simulink model "pwaSys_obs_model_ud"  (Simulink 8.6)
settings: Solver=ode45  StartTime=0.0  StopTime=sim_T  RelTol=1e-3
InitFcn:
  | load simulink.mat
  | setParameters
StartFcn:
  | load simulink.mat
  | setParameters
  | clear res_X res_U res_Y res_P res_D
  | clear res_Xest res_Dest res_Yest
StopFcn:
  | plotScope
undefined symbols (not defined in the file): sigbuilder_block, sim_A, sim_B, sim_C, sim_D, sim_d, sim_d_scale_bias, sim_d_scale_gain, sim_H, sim_K, sim_nx, sim_ny, sim_Ts, sim_u, sim_u_scale_bias, sim_u_scale_gain, sim_x0, sim_x_scale_bias, sim_x_scale_gain, sim_y_scale_bias, sim_y_scale_gain
libraries: xbsIndex_r4 x8
settings Model: Creator=alberto  LastModifiedBy=matteo
settings DataIOCC: SignalLoggingSaveFormat=Dataset
settings OptimizationCC: ExpressionDepthLimit=128
settings DebuggingCC: UnderspecifiedInitializationDetection=Simplified  MergeDetectMultiDrivingBlocksExec=error  FcnCallInpInsideContextMsg=EnableAllAsError  StateNameClashWarn=none
settings GRTTargetCC: CombineOutputUpdateFcns=on  GRTInterface=off
settings ConfigComp: CovSFcnEnable=off

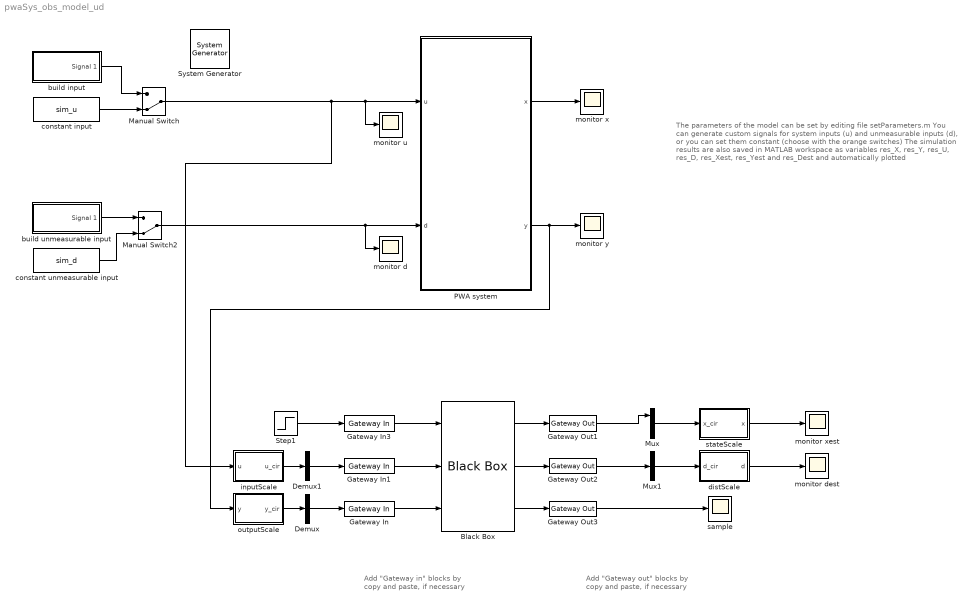
== system pwaSys_obs_model_ud ==
  note: The parameters of the model can be set by editing file setParameters.m
      |
      | You can generate custom signals for system inputs (u) and unmeasurable
      | inputs (d), or you can set them constant (choose with the orange switches)
      |
      | The simulation results are also saved in MATLAB workspace as variables
      | res_X, res_Y, res_U, res_D, res_Xest, res_Yest and res_Dest and
      | automatically plotted
  note: Add "Gateway out" blocks
      | by copy and paste,
      | if necessary
  note: Add "Gateway in" blocks
      | by copy and paste,
      | if necessary
  " System Generator" : xbsIndex_r4/ System Generator  Tag=genX  xilinxfamily=kintex7  part=xc7k325t  speed=-3  package=fbg676  synthesis_tool=Vivado  clock_wrapper=Clock Enables  directory=./netlist  proj_type=Vivado  Synth_file=Vivado Synthesis Defaults  Impl_file=Vivado Implementation Defaults  testbench=off  simulink_period=clk_period  sysclk_period=10  dcm_input_clock_period=10  incr_netlist=off  trim_vbits=Everywhere in SubSystem  dbl_ovrd=According to Block Masks  core_generation=According to Block Masks  run_coregen=off  deprecated_control=off  eval_field=0  block_type=sysgen
  Black Box : xbsIndex_r4/Black Box  init_code=embeddedSystem_config  sim_method=ISE Simulator  verbose=off  block_type=blackbox2
  Demux : Demux  Outputs=sim_ny
  Demux1 : Demux  Outputs=sim_nu
  Gateway In : xbsIndex_r4/Gateway In  gui_display_data_type=Fixed-point  arith_type="Signed  (2's comp)"  n_bits=sim_n_bit_in  bin_pt=0  preci_type=Single  exp_width=8  frac_width=24  rows=1  columns=1  quantization="Round  (unbiased: +/- Inf)"  overflow=Saturate  period=clk_period  UseAsADC=off  ADCChannel='1'  interface=None  automatic_assignment=on  address_offset=hex2dec('00')  intf_name=''  intf_description=''  timing_constraint=None  locs_specified=off  LOCs={}  io_standard={}  inherit_from_input=off  hdl_port=on  dbl_ovrd=off  block_type=gatewayin
  Gateway In1 : xbsIndex_r4/Gateway In  gui_display_data_type=Fixed-point  arith_type="Signed  (2's comp)"  n_bits=sim_n_bit_in  bin_pt=0  preci_type=Single  exp_width=8  frac_width=24  rows=1  columns=1  quantization="Round  (unbiased: +/- Inf)"  overflow=Saturate  period=clk_period  UseAsADC=off  ADCChannel='1'  interface=None  automatic_assignment=on  address_offset=hex2dec('00')  intf_name=''  intf_description=''  timing_constraint=None  locs_specified=off  LOCs={}  io_standard={}  inherit_from_input=off  hdl_port=on  dbl_ovrd=off  block_type=gatewayin
  Gateway In3 : xbsIndex_r4/Gateway In  gui_display_data_type=Boolean  arith_type=Boolean  n_bits=16  bin_pt=14  preci_type=Single  exp_width=8  frac_width=24  rows=1  columns=1  quantization="Round  (unbiased: +/- Inf)"  overflow=Saturate  period=clk_period  UseAsADC=off  ADCChannel='1'  interface=None  automatic_assignment=on  address_offset=hex2dec('00')  intf_name=''  intf_description=''  timing_constraint=None  locs_specified=off  LOCs={}  io_standard={}  inherit_from_input=off  hdl_port=on  dbl_ovrd=off  block_type=gatewayin
  Gateway Out1 : xbsIndex_r4/Gateway Out  inherit_from_input=off  hdl_port=on  rows=1  columns=1  UseAsDAC=off  DACChannel='1'  interface=None  automatic_assignment=on  address_offset=hex2dec('00')  intf_name=''  intf_description=''  timing_constraint=None  locs_specified=off  LOCs={}  io_standard={}  block_type=gatewayout
  Gateway Out2 : xbsIndex_r4/Gateway Out  inherit_from_input=off  hdl_port=on  rows=1  columns=1  UseAsDAC=off  DACChannel='1'  interface=None  automatic_assignment=on  address_offset=hex2dec('00')  intf_name=''  intf_description=''  timing_constraint=None  locs_specified=off  LOCs={}  io_standard={}  block_type=gatewayout
  Gateway Out3 : xbsIndex_r4/Gateway Out  inherit_from_input=off  hdl_port=on  rows=1  columns=1  UseAsDAC=off  DACChannel='1'  interface=None  automatic_assignment=on  address_offset=hex2dec('00')  intf_name=''  intf_description=''  timing_constraint=None  locs_specified=off  LOCs={}  io_standard={}  block_type=gatewayout
  Manual Switch : ManualSwitch  CurrentSetting=0
  Manual Switch2 : ManualSwitch  CurrentSetting=0
  Mux : Mux  Inputs=sim_nx
  Mux1 : Mux  Inputs=sim_nd
  PWA system : Subsystem
  Step1 : Step  Time=0.5  SampleTime=0
  build input : Subsystem  Tag=STV Subsys  LoadFcn=sigbuilder_block('load');  StartFcn=sigbuilder_block('start');  StopFcn=sigbuilder_block('stop');  ClipboardFcn=sigbuilder_block('clipboard');  mask(Sigbuilder block){}
      mask help: Simulink:masks:SigbuilderBlock_MD
      mask init:
      | if ~strcmp(get_param(bdroot(gcbh),'SimulationStatus'),'stopped') tuvar = sigbuilder_block('maskInit'); end
      settings: CopyFcn=sigbuilder_block('copy');  DeleteFcn=sigbuilder_block('delete');  ModelCloseFcn=sigbuilder_block('modelClose');  PreSaveFcn=sigbuilder_block('preSave');  PauseFcn=sigbuilder_block('pause');  ContinueFcn=sigbuilder_block('continue');  NameChangeFcn=sigbuilder_block('namechange');  OpenFcn=sigbuilder_block('open',[433.6 120 558.4 400.8 ]);  CloseFcn=sigbuilder_block('close');
      mask Display: plot(0, 0, 100, 100,[2, 2, 32, 32, 2], [68, 8, 8, 68, 68],[32, 2], [38, 38], [32, 19, 2],[53, 60, 44], [32, 17, 17, 2],[16, 16, 31, 31]);txt = getActiveGroup(gcbh);text(2, 100, txt,'verticalAlignment', 'top');
  build unmeasurable input : Subsystem  Tag=STV Subsys  LoadFcn=sigbuilder_block('load');  StartFcn=sigbuilder_block('start');  StopFcn=sigbuilder_block('stop');  ClipboardFcn=sigbuilder_block('clipboard');  mask(Sigbuilder block){}
      mask help: Simulink:masks:SigbuilderBlock_MD
      mask init:
      | if ~strcmp(get_param(bdroot(gcbh),'SimulationStatus'),'stopped') tuvar = sigbuilder_block('maskInit'); end
      settings: CopyFcn=sigbuilder_block('copy');  DeleteFcn=sigbuilder_block('delete');  ModelCloseFcn=sigbuilder_block('modelClose');  PreSaveFcn=sigbuilder_block('preSave');  PauseFcn=sigbuilder_block('pause');  ContinueFcn=sigbuilder_block('continue');  NameChangeFcn=sigbuilder_block('namechange');  OpenFcn=sigbuilder_block('open',[433.6 121.6 550.4 399.2 ]);  CloseFcn=sigbuilder_block('close');
      mask Display: plot(0, 0, 100, 100,[2, 2, 32, 32, 2], [68, 8, 8, 68, 68],[32, 2], [38, 38], [32, 19, 2],[53, 60, 44], [32, 17, 17, 2],[16, 16, 31, 31]);txt = getActiveGroup(gcbh);text(2, 100, txt,'verticalAlignment', 'top');
  constant input : Constant  Value=sim_u
  constant unmeasurable input : Constant  Value=sim_d
  "distScale " : Subsystem
  inputScale : Subsystem
  monitor d : Scope
  monitor dest : Scope
  monitor u : Scope
  monitor x : Scope
  monitor xest : Scope
  monitor y : Scope
  outputScale : Subsystem
  sample : Scope
  stateScale : Subsystem
  wires:
  PWA system/1(x) -> monitor x/1
  build unmeasurable input/1(Signal 1) -> Manual Switch2/1
  constant unmeasurable input/1 -> Manual Switch2/2
  Manual Switch2/1 -> monitor d/1, PWA system/2(d)
  build input/1(Signal 1) -> Manual Switch/1
  constant input/1 -> Manual Switch/2
  stateScale/1("x ") -> monitor xest/1
  PWA system/2(y) -> outputScale/1(y), monitor y/1
  outputScale/1("y_cir ") -> Demux/1
  Gateway In3/1 -> Black Box/1
  Step1/1 -> Gateway In3/1
  Demux/1 -> Gateway In/1
  Gateway In/1 -> Black Box/3
  Black Box/1 -> Gateway Out1/1
  Gateway Out3/1 -> sample/1
  Gateway Out1/1 -> Mux/1
  Mux/1 -> stateScale/1(x_cir)
  Black Box/3 -> Gateway Out3/1
  "distScale "/1("d ") -> monitor dest/1
  Black Box/2 -> Gateway Out2/1
  Gateway Out2/1 -> Mux1/1
  Mux1/1 -> "distScale "/1(d_cir)
  Manual Switch/1 -> inputScale/1(u), monitor u/1, PWA system/1(u)
  inputScale/1("u_cir ") -> Demux1/1
  Demux1/1 -> Gateway In1/1
  Gateway In1/1 -> Black Box/2

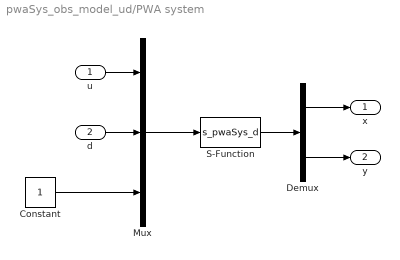
== system pwaSys_obs_model_ud/PWA system ==
  u : Inport
  d : Inport  Port=2
  Constant : Constant
  Demux : Demux  Outputs=[sim_nx sim_ny]
  Mux : Mux  Inputs=3
  S-Function : S-Function  FunctionName=s_pwaSys_d  Parameters=A,B,C,D,H,K,sim_x0,Ts  SFunctionDeploymentMode=off  EnableBusSupport=off  mask{A=sim_A, B=sim_B, C=sim_C, D=sim_D, H=sim_H, K=sim_K, sim_x0=sim_x0, Ts=sim_Ts}
      mask prompts: sim_x0 "Initial condition"; Ts "Sample time"
      mask DialogControl DescTextVar Prompt: continuous time PWA system
  x : Outport
  y : Outport  Port=2
  wires:
  u/1 -> Mux/1
  Mux/1 -> S-Function/1
  S-Function/1 -> Demux/1
  Demux/1 -> x/1
  Demux/2 -> y/1
  Constant/1 -> Mux/3
  d/1 -> Mux/2

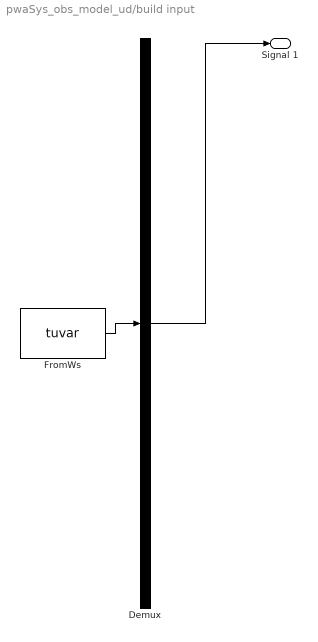
== system pwaSys_obs_model_ud/build input ==
  Demux : Demux  Tag=STV Demux  Outputs=1
  FromWs : FromWorkspace  Tag=STV FromWs  VariableName=tuvar  SampleTime=0  SigBuilderData=DataTag1  VnvData=DataTag2
      SigBuilderData=|
      | common.afterFinalStr = 'Extrapolate'
      | common.sampleTime = 0
      | dataSet.timeRange = [0 10]
      | dataSet.name = 'Group 1'
      | sbobj.Groups.Name = 'Group 1'
      | sbobj.Groups.Signals.Name = 'Signal 1'
      | sbobj.Groups.Signals.XData = [0 6 10]
      | sbobj.Groups.Signals.YData = [0 0 0]
  Signal 1 : Outport  Tag=STV Outport
  wires:
  Demux/1 -> Signal 1/1
  FromWs/1 -> Demux/1

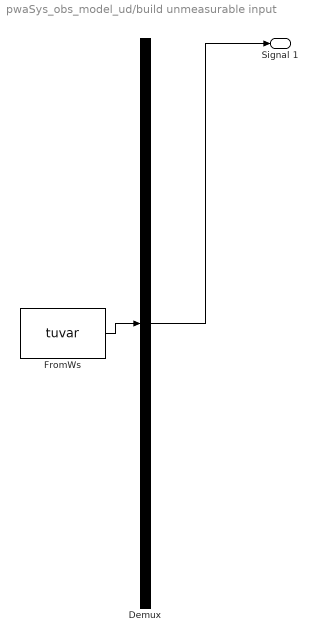
== system pwaSys_obs_model_ud/build unmeasurable input ==
  Demux : Demux  Tag=STV Demux  Outputs=1
  FromWs : FromWorkspace  Tag=STV FromWs  VariableName=tuvar  SampleTime=0  SigBuilderData=DataTag3  VnvData=DataTag4
      SigBuilderData=|
      | common.afterFinalStr = 'Extrapolate'
      | common.sampleTime = 0
      | dataSet.timeRange = [0 10]
      | dataSet.name = 'Group 1'
      | sbobj.Groups.Name = 'Group 1'
      | sbobj.Groups.Signals.Name = 'Signal 1'
      | sbobj.Groups.Signals.XData = [0 6 10]
      | sbobj.Groups.Signals.YData = [0 0 0]
  Signal 1 : Outport  Tag=STV Outport
  wires:
  Demux/1 -> Signal 1/1
  FromWs/1 -> Demux/1

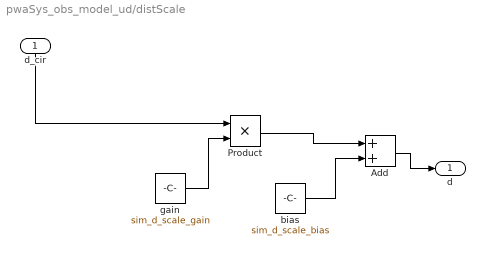
== system pwaSys_obs_model_ud/distScale  ==
  d_cir : Inport
  Add : Sum
  Product : Product
  bias : Constant  Value=sim_d_scale_bias
  gain : Constant  Value=sim_d_scale_gain
  "d " : Outport
  wires:
  bias/1 -> Add/2
  gain/1 -> Product/2
  Add/1 -> "d "/1
  d_cir/1 -> Product/1
  Product/1 -> Add/1

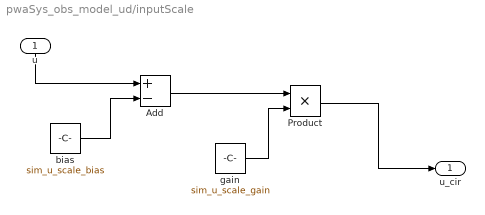
== system pwaSys_obs_model_ud/inputScale ==
  u : Inport
  Add : Sum  Inputs=+-
  Product : Product
  bias : Constant  Value=sim_u_scale_bias
  gain : Constant  Value=sim_u_scale_gain
  "u_cir " : Outport
  wires:
  Product/1 -> "u_cir "/1
  bias/1 -> Add/2
  u/1 -> Add/1
  Add/1 -> Product/1
  gain/1 -> Product/2

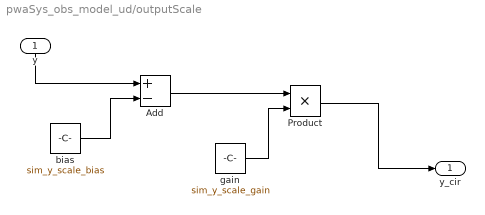
== system pwaSys_obs_model_ud/outputScale ==
  y : Inport
  Add : Sum  Inputs=+-
  Product : Product
  bias : Constant  Value=sim_y_scale_bias
  gain : Constant  Value=sim_y_scale_gain
  "y_cir " : Outport
  wires:
  Product/1 -> "y_cir "/1
  bias/1 -> Add/2
  y/1 -> Add/1
  Add/1 -> Product/1
  gain/1 -> Product/2

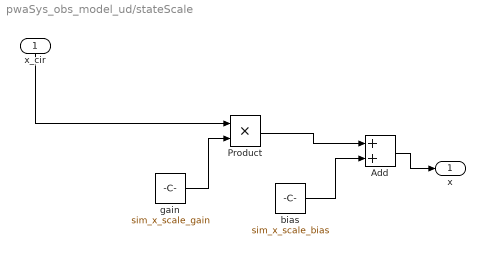
== system pwaSys_obs_model_ud/stateScale ==
  x_cir : Inport
  Add : Sum
  Product : Product
  bias : Constant  Value=sim_x_scale_bias
  gain : Constant  Value=sim_x_scale_gain
  "x " : Outport
  wires:
  bias/1 -> Add/2
  gain/1 -> Product/2
  Add/1 -> "x "/1
  x_cir/1 -> Product/1
  Product/1 -> Add/1
